simulink model "hiv_model_ekf_template"  (R2019b)
settings: Solver=VariableStepAuto  StartTime=0.0  StopTime=10.0  RelTol=1e-3
values from neighbouring files (symbols this model uses):
  Delta = 0.01    [init.m]
  Theta = block.DialogPrm(2).Data    [hiv_model.m]    (also in init.m = [0.25 50 0.25 10 0.01 0.0045]')
  xdash0 = [1000 550 0.0001]'    [init.m]
  xdash12RL = block.DialogPrm(3).Data    [hiv_model.m]    (also in init.m = [1000 550]')
settings Model: Creator=schauer  LastModifiedBy=schauer

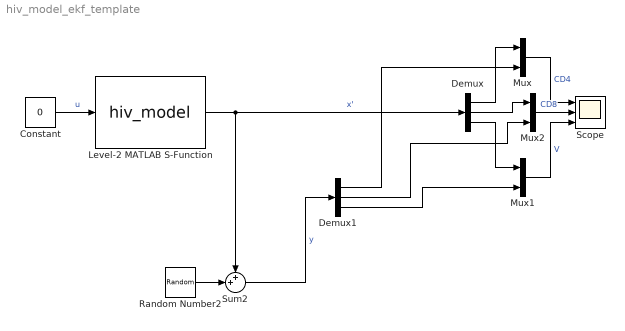
== system hiv_model_ekf_template ==
  Constant : Constant  Value=0
  Demux : Demux  Outputs=3
  Demux1 : Demux  Outputs=3
  Level-2 MATLAB S-Function : M-S-Function  FunctionName=hiv_model  Parameters=xdash0,Theta,xdash12RL
  Mux : Mux  Inputs=2
  Mux1 : Mux  Inputs=2
  Mux2 : Mux  Inputs=2
  Random Number2 : RandomNumber  Variance=[100 100 10^-5]  SampleTime=Delta
  Scope : Scope  NumInputPorts=3
  Sum2 : Sum  Inputs=++|
  wires:
  Constant/1 -> Level-2 MATLAB S-Function/1  "u"
  Level-2 MATLAB S-Function/1 -> Demux/1, Sum2/1  "x'"
  Mux/1 -> Scope/1  "CD4"
  Demux/1 -> Mux/1
  Demux/3 -> Mux1/1
  Mux1/1 -> Scope/3  "V"
  Sum2/1 -> Demux1/1  "y"
  Random Number2/1 -> Sum2/2
  Mux2/1 -> Scope/2  "CD8"
  Demux/2 -> Mux2/1
  Demux1/1 -> Mux/2
  Demux1/2 -> Mux2/2
  Demux1/3 -> Mux1/2
